simulink subsystem "ApplicationAbstractionOpenLoop"  (R2024b)
settings: Solver=VariableStepAuto  StartTime=0.0  StopTime=10.0  RelTol=1e-3
undefined symbols (not defined in the file or in its folder): pmsm
libraries: mcbpositiondecoderlib x6, mcbcontrolslib x2
settings Model: Creator=The MathWorks, Inc.  LastModifiedBy=The MathWorks, Inc.
settings RTWCC: GPUComputeCapability=3.5  LargeConstantGeneration=WriteOnlyDNNConstantsToDataFiles

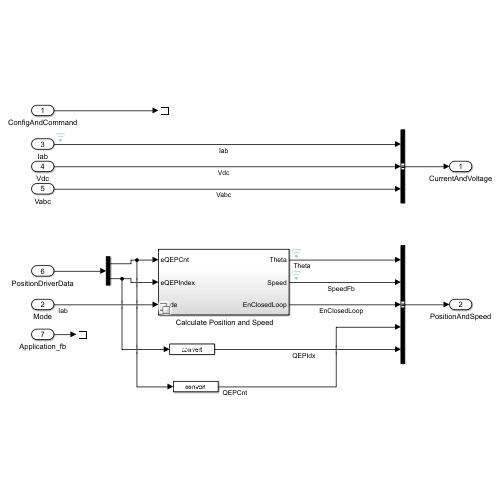
[thumbnail: Simulink's stored preview of the top-level diagram]
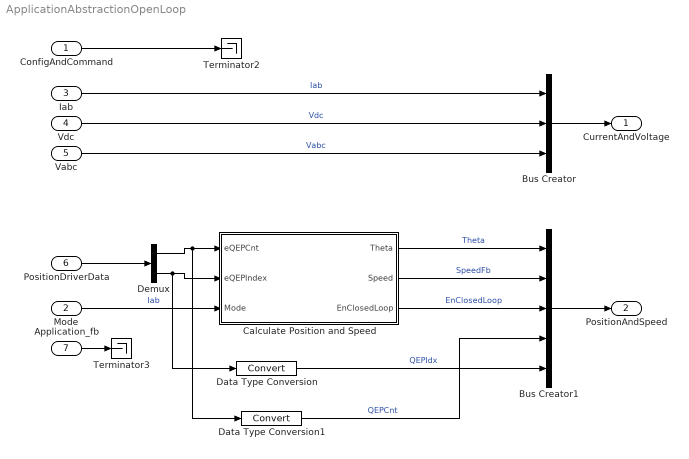
== system ApplicationAbstractionOpenLoop ==
  ConfigAndCommand : Inport
  Mode : Inport  Port=2
  Iab : Inport  Port=3
  Vdc : Inport  Port=4
  Vabc : Inport  Port=5
  PositionDriverData : Inport  Port=6
  Application_fb : Inport  Port=7
  " Calculate Position and Speed" : Subsystem  Variant=on
  Bus Creator : BusCreator  Inputs=3
  Bus Creator1 : BusCreator  Inputs=5
  Data Type Conversion : DataTypeConversion  SaturateOnIntegerOverflow=off  RndMeth=Floor
  Data Type Conversion1 : DataTypeConversion  SaturateOnIntegerOverflow=off  RndMeth=Floor
  Demux : Demux  Outputs=2
  Terminator2 : Terminator
  Terminator3 : Terminator
  CurrentAndVoltage : Outport
  PositionAndSpeed : Outport  Port=2
  wires:
  PositionDriverData/1 -> Demux/1
  Bus Creator/1 -> CurrentAndVoltage/1
  Iab/1 -> Bus Creator/1  "Iab"
  " Calculate Position and Speed"/2(Speed) -> Bus Creator1/2  "SpeedFb"
  " Calculate Position and Speed"/1(Theta) -> Bus Creator1/1  "Theta"
  Bus Creator1/1 -> PositionAndSpeed/1
  ConfigAndCommand/1 -> Terminator2/1
  Demux/1 -> " Calculate Position and Speed"/1(eQEPCnt), Data Type Conversion1/1
  Demux/2 -> " Calculate Position and Speed"/2(eQEPIndex), Data Type Conversion/1
  " Calculate Position and Speed"/3(EnClosedLoop) -> Bus Creator1/3  "EnClosedLoop"
  Mode/1 -> " Calculate Position and Speed"/3(Mode)  "Iab"
  Application_fb/1 -> Terminator3/1
  Vdc/1 -> Bus Creator/2  "Vdc"
  Vabc/1 -> Bus Creator/3  "Vabc"
  Data Type Conversion/1 -> Bus Creator1/5  "QEPIdx"
  Data Type Conversion1/1 -> Bus Creator1/4  "QEPCnt"

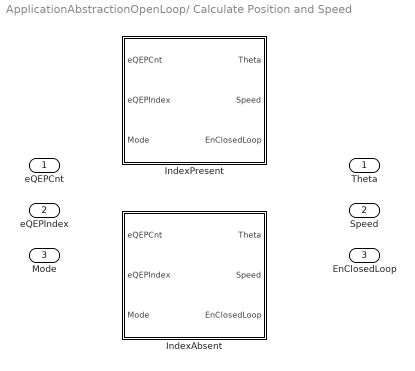
== system ApplicationAbstractionOpenLoop/ Calculate Position and Speed ==
  eQEPCnt : Inport
  eQEPIndex : Inport  Port=2
  Mode : Inport  Port=3
  IndexAbsent : Subsystem  VariantControl=pmsm.QEPIndexPresent == false
  IndexPresent : Subsystem  VariantControl=pmsm.QEPIndexPresent == true
  Theta : Outport
  Speed : Outport  Port=2
  EnClosedLoop : Outport  Port=3

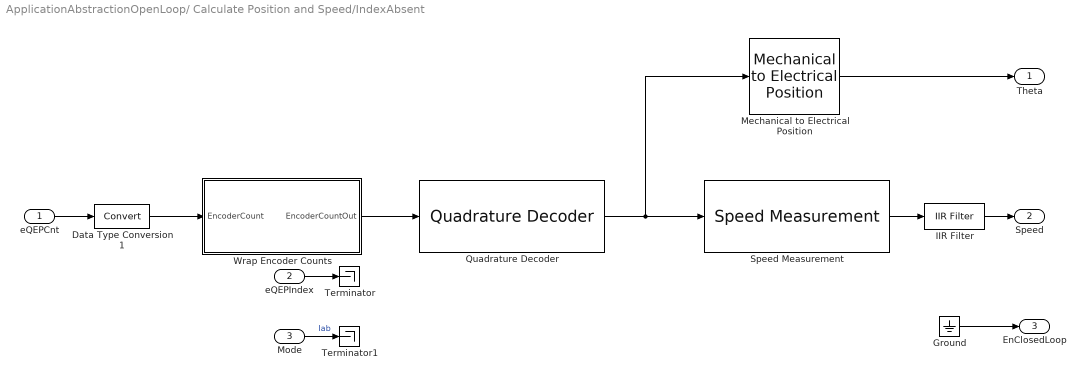
== system ApplicationAbstractionOpenLoop/ Calculate Position and Speed/IndexAbsent ==
  eQEPCnt : Inport
  eQEPIndex : Inport  Port=2
  Mode : Inport  Port=3
  Data Type Conversion1 : DataTypeConversion  RndMeth=Simplest  SaturateOnIntegerOverflow=off
  Ground : Ground
  IIR Filter : mcbcontrolslib/IIR Filter  VariantControl=Low Pass Filter  VariantSelect=Low-pass  FilterConstantInputType=Specify via dialog  Filter_constant=0.01  advancedSettings=off  Ts=50e-6  cutOff_freq=32.1525
  Mechanical to Electrical Position : mcbpositiondecoderlib/Mechanical to Electrical Position  PolePairsInputType=Specify via dialog  NrPP=pmsm.p  selectedRange=Radians  MechOfstInputType=Specify via dialog  mechOffsetIn=pmsm.PositionOffset  maxAngleIn=2*pi  InputDataType=dataType  VariantSelect=floating-point
  Quadrature Decoder : mcbpositiondecoderlib/Quadrature Decoder  EncoderSlitsPerRevolution=pmsm.QEPSlits  EncoderCountsPerSlit=4  CounterSize=16 bits  ExternalIndexCount=off  PositionUnit=Radians  PositionDataType=dataType  ParameterInputType=off  CountsPerRevInverseDataType=single
  Speed Measurement : mcbpositiondecoderlib/Speed Measurement  PositionUnit=Radians  PositionScalingDatatype=uint32  SpeedCalculationMode=Time interval for speed calculation  SampleTimeAsync=Ts  MaximumApplicationSpeed=6000  SpeedResolution=5e-6  DelayLength=20  MaximumMeasurableSpeed=-0.98352  MeasurableSpeedResolution=7.6757e-12  SpeedUnit=RPM  PerUnitSpeed=PU_System.N_base  SpeedDataType=dataType
  Terminator : Terminator
  Terminator1 : Terminator
  Wrap Encoder Counts : Subsystem  mask{EnCountPerRev=pmsm.QEPSlits*4}
      mask prompts: EnCountPerRev "Encoder counts per rev"
  Theta : Outport
  Speed : Outport  Port=2
  EnClosedLoop : Outport  Port=3
  wires:
  eQEPCnt/1 -> Data Type Conversion1/1
  Data Type Conversion1/1 -> Wrap Encoder Counts/1(EncoderCount)
  Mode/1 -> Terminator1/1  "Iab"
  Ground/1 -> EnClosedLoop/1
  IIR Filter/1 -> Speed/1
  Mechanical to Electrical Position/1 -> Theta/1
  eQEPIndex/1 -> Terminator/1
  Speed Measurement/1 -> IIR Filter/1
  Quadrature Decoder/1 -> Mechanical to Electrical Position/1, Speed Measurement/1
  Wrap Encoder Counts/1(EncoderCountOut) -> Quadrature Decoder/1

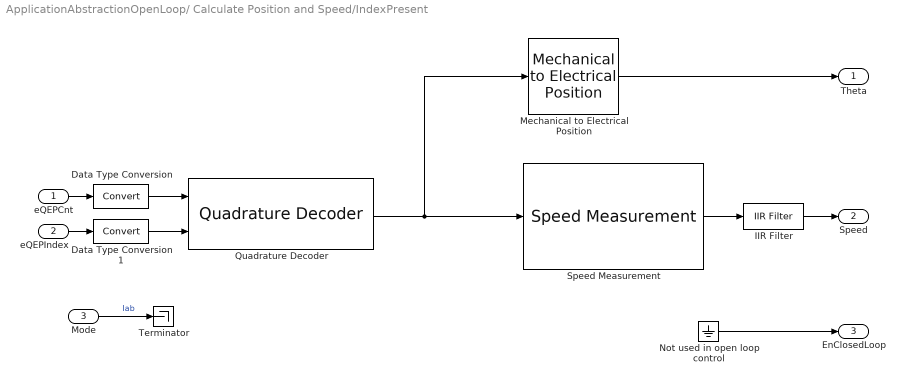
== system ApplicationAbstractionOpenLoop/ Calculate Position and Speed/IndexPresent ==
  eQEPCnt : Inport
  eQEPIndex : Inport  Port=2
  Mode : Inport  Port=3
  Data Type Conversion : DataTypeConversion  RndMeth=Simplest  SaturateOnIntegerOverflow=off
  Data Type Conversion1 : DataTypeConversion  RndMeth=Simplest  SaturateOnIntegerOverflow=off
  IIR Filter : mcbcontrolslib/IIR Filter  VariantControl=Low Pass Filter  VariantSelect=Low-pass  FilterConstantInputType=Specify via dialog  Filter_constant=0.01  advancedSettings=off  Ts=50e-6  cutOff_freq=32.1525
  Mechanical to Electrical Position : mcbpositiondecoderlib/Mechanical to Electrical Position  PolePairsInputType=Specify via dialog  NrPP=pmsm.p  selectedRange=Radians  MechOfstInputType=Specify via dialog  mechOffsetIn=pmsm.PositionOffset  maxAngleIn=2*pi  InputDataType=dataType  VariantSelect=floating-point
  Not used in open loop control : Ground
  Quadrature Decoder : mcbpositiondecoderlib/Quadrature Decoder  EncoderSlitsPerRevolution=pmsm.QEPSlits  EncoderCountsPerSlit=4  CounterSize=16 bits  ExternalIndexCount=on  PositionUnit=Radians  PositionDataType=dataType  ParameterInputType=off  CountsPerRevInverseDataType=single
  Speed Measurement : mcbpositiondecoderlib/Speed Measurement  PositionUnit=Radians  PositionScalingDatatype=uint32  SpeedCalculationMode=Time interval for speed calculation  SampleTimeAsync=Ts  MaximumApplicationSpeed=6000  SpeedResolution=5e-6  DelayLength=20  MaximumMeasurableSpeed=-0.98352  MeasurableSpeedResolution=7.6757e-12  SpeedUnit=RPM  PerUnitSpeed=PU_System.N_base  SpeedDataType=dataType
  Terminator : Terminator
  Theta : Outport
  Speed : Outport  Port=2
  EnClosedLoop : Outport  Port=3
  wires:
  Data Type Conversion1/1 -> Quadrature Decoder/2
  Data Type Conversion/1 -> Quadrature Decoder/1
  Mode/1 -> Terminator/1  "Iab"
  Not used in open loop control/1 -> EnClosedLoop/1
  IIR Filter/1 -> Speed/1
  eQEPIndex/1 -> Data Type Conversion1/1
  Speed Measurement/1 -> IIR Filter/1
  eQEPCnt/1 -> Data Type Conversion/1
  Mechanical to Electrical Position/1 -> Theta/1
  Quadrature Decoder/1 -> Mechanical to Electrical Position/1, Speed Measurement/1

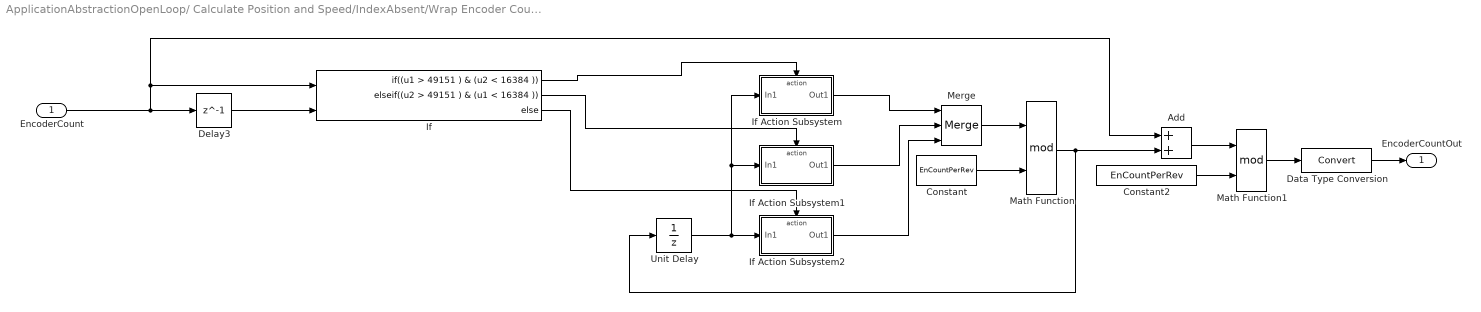
== system ApplicationAbstractionOpenLoop/ Calculate Position and Speed/IndexAbsent/Wrap Encoder Counts ==
  EncoderCount : Inport
  Add : Sum  OutDataTypeStr=single
  Constant : Constant  Value=EnCountPerRev  OutDataTypeStr=Inherit: Inherit via back propagation
  Constant2 : Constant  Value=EnCountPerRev  OutDataTypeStr=Inherit: Inherit via back propagation
  Data Type Conversion : DataTypeConversion  RndMeth=Simplest  SaturateOnIntegerOverflow=off
  Delay3 : Delay  DelayLength=1  InitialCondition=0
  If : If  NumInputs=2  IfExpression=(u1 > 49151 ) & (u2 < 16384 )  ElseIfExpressions=(u2 > 49151 ) & (u1 < 16384 )
  If Action Subsystem : Subsystem  TreatAsAtomicUnit=on
  If Action Subsystem1 : Subsystem  TreatAsAtomicUnit=on
  If Action Subsystem2 : Subsystem  TreatAsAtomicUnit=on
  Math Function : Math  Operator=mod  SignedPower=on
  Math Function1 : Math  Operator=mod  SignedPower=on
  Merge : Merge  Inputs=3
  Unit Delay : UnitDelay  SampleTime=-1  HasFrameUpgradeWarning=on
  EncoderCountOut : Outport
  wires:
  EncoderCount/1 -> Add/1, If/1, Delay3/1
  If Action Subsystem2/1(Out1) -> Merge/3
  If/2 -> If Action Subsystem1/Action
  If Action Subsystem1/1(Out1) -> Merge/2
  Unit Delay/1 -> If Action Subsystem/1(In1), If Action Subsystem1/1(In1), If Action Subsystem2/1(In1)
  If/3 -> If Action Subsystem2/Action
  If Action Subsystem/1(Out1) -> Merge/1
  Constant/1 -> Math Function/2
  Delay3/1 -> If/2
  Merge/1 -> Math Function/1
  If/1 -> If Action Subsystem/Action
  Math Function/1 -> Unit Delay/1, Add/2
  Add/1 -> Math Function1/1
  Constant2/1 -> Math Function1/2
  Math Function1/1 -> Data Type Conversion/1
  Data Type Conversion/1 -> EncoderCountOut/1

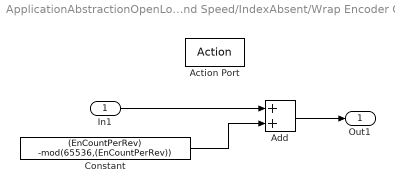
== system ApplicationAbstractionOpenLoop/ Calculate Position and Speed/IndexAbsent/Wrap Encoder Counts/If Action Subsystem ==
  In1 : Inport
  Action Port : ActionPort
  Add : Sum
  Constant : Constant  Value=(EnCountPerRev) -mod(65536,(EnCountPerRev))  OutDataTypeStr=uint16
  Out1 : Outport
  wires:
  In1/1 -> Add/1
  Constant/1 -> Add/2
  Add/1 -> Out1/1

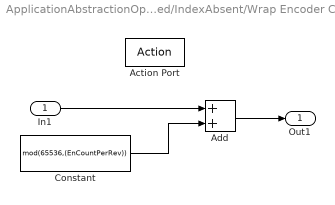
== system ApplicationAbstractionOpenLoop/ Calculate Position and Speed/IndexAbsent/Wrap Encoder Counts/If Action Subsystem1 ==
  In1 : Inport
  Action Port : ActionPort
  Add : Sum
  Constant : Constant  Value=mod(65536,(EnCountPerRev))  OutDataTypeStr=uint16
  Out1 : Outport
  wires:
  Add/1 -> Out1/1
  Constant/1 -> Add/2
  In1/1 -> Add/1

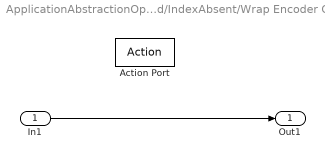
== system ApplicationAbstractionOpenLoop/ Calculate Position and Speed/IndexAbsent/Wrap Encoder Counts/If Action Subsystem2 ==
  In1 : Inport
  Action Port : ActionPort
  Out1 : Outport
  wires:
  In1/1 -> Out1/1
